simulink model "pipe_strat_enhanced"  (R2018b)
settings: Solver=VariableStepAuto  StartTime=0.0  StopTime=10.0  RelTol=1e-3
undefined symbols (not defined in the file): nodes
libraries: simulink x5, carnot x1
settings Model: Creator=jonas.gottschald  LastModifiedBy=P41573
settings DataIOCC: ReturnWorkspaceOutputs=on

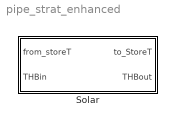
== system pipe_strat_enhanced ==
  Solar : Subsystem  AncestorBlock=carnot/Storage/Thermal/Storage_Ports/Pipe_stratified  mask(pipe connection to storage){h_in=1, h_strat=0.16, h_out=0, hgt=1, dia=0.08, height=-1, nodes=nodes}
      mask prompts: h_in "relative height of the starting point of the stratification device"; h_strat "relative height of the end point of the stratification device"; h_out "relative height of outlet"; hgt "Height of storage in m"; dia "Diameter of pipe in m"; height "Height difference inlet-outlet"; nodes "Number of nodes (DO NOT CHANGE)"
      mask help:
      | The block transforms the incoming THV vector to a vector which the storage interprets as a flow into the storage fluid.
      | Give inlet- and outlet-height as a relative position from 0 (= bottom) to 1 (= top).
      mask init:
      | in = zeros(nodes,1);    % vector of length nodes
      | up = in;                % vector of length nodes
      | down = in;              % vector of length nodes
      | 
      | h_in = max(0,min(h_in,1));     % no nodes below 0 and above 1
      | h_out = max(0,min(h_out,1));   % no nodes below 0 and above 1
      | h_strat = max(0,min(h_strat,1));   % no nodes below 0 and above 1
      | set_param(gcb,'height',num2str((h_out-h_in)*hgt));
      | 
      | inlet = max(ceil(h_in*nodes),1);    % inlet position
      | outlet = max(ceil(h_out*nodes),1);  % outlet position
      | strat = max(ceil(h_strat*nodes),1);  % startification position
      | hgt = (h_out-h_in)*hgt;
      | in(inlet)=1;
      | 
      | idx_in_out = inlet:outlet;
      | if (inlet < outlet && strat < outlet && inlet < strat)      % if outlet above inlet and stratification and inlet below stratification
      |     up(inlet:outlet-1)=1;       % upwards
      |     n_concerned = inlet:strat;
      | end
      | 
      | if (inlet < outlet && strat < outlet && inlet > strat) % if outlet above inlet and stratification and inlet above stratification
      |     up(strat:outlet-1)=1;       % upwards
      |     n_concerned = strat:inlet;
      | end
      | 
      | if (inlet < outlet && strat > outlet)                  % if outlet above inlet and below stratification
      |     up(inlet:outlet-1)=1;       % upwards and
      |     down(outlet:strat-1)=1;     % downwards
      |     n_concerned = inlet:strat;
      | end
      | 
      | if (inlet > outlet && strat < outlet)                  % if outlet below inlet and above stratification
      |     up(strat:outlet-1)=1;       % upwars and
      |     down(outlet:inlet-1)=1;     % downwards
      |     n_concerned = strat:inlet;
      |     idx_in_out = outlet:inlet;
      | end
      | 
      | if (inlet > outlet && inlet > strat)                    % if inlet above outlet and above stratification
      |     down(outlet:inlet-1)=1;     % downwards
      |     n_concerned = strat:inlet;                              % if inlet above outlet and below stratification
      |     idx_in_out = outlet:inlet;
      | end
      | 
      | if (inlet > outlet && inlet < strat)
      |     down(outlet:strat-1)=1;     % downwards
      |     n_concerned = inlet:strat;
      |     idx_in_out = outlet:inlet;
      | end
      mask Help: web(fullfile(path_carnot('help'),'StoragePorts_PipeConnections.html'),'-helpbrowser')
      mask TypeOptions dia: Pressure_Drop_StoragePipe/dia
      mask TypeOptions height: Pressure_Drop_StoragePipe/hgt
      mask DialogControl ParameterTabVar0 Prompt: Geometry
      mask DialogControl ParameterTabVar02 Prompt: Calculation
      mask Display: disp('Pipe STRAT')

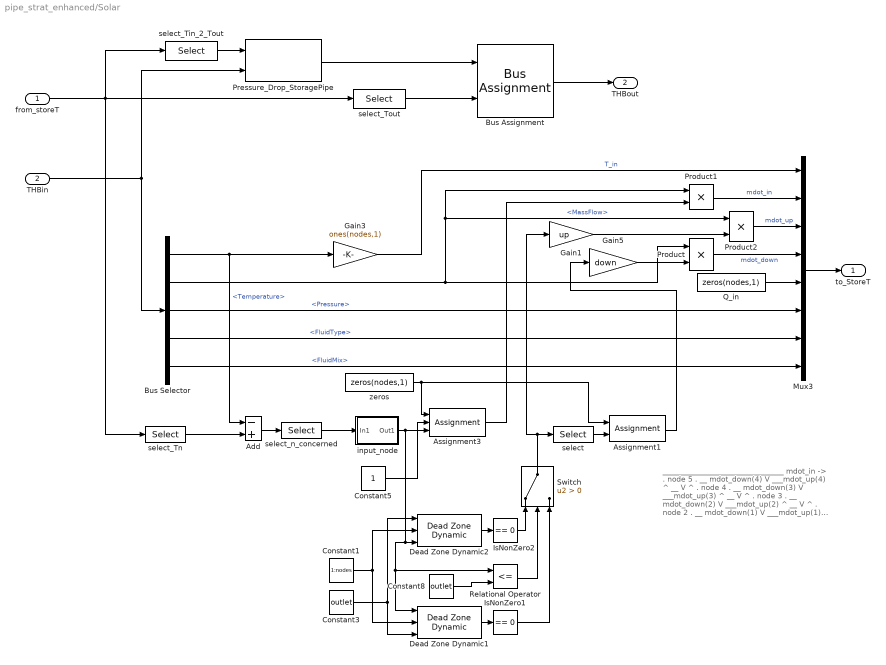
== system pipe_strat_enhanced/Solar ==
  note: _________________________________
      | mdot_in ->                                                .
      | node 5                     .
      | __ mdot_down(4) V  ___mdot_up(4) ^ __
      | V                           ^    .
      | node 4                    .
      | __ mdot_down(3) V  ___mdot_up(3) ^ __
      | V                           ^    .
      | node 3                    .
      | __ mdot_down(2) V  ___mdot_up(2) ^ __
      | V                           ^    .
      | node 2                    .
      | __ mdot_down(1) V  ___mdot_up(1) ^ __
      | V                           ^    .
      | node 1                    .
      | _________________________________
  from_storeT : Inport
  THBin : Inport  Port=2
  Add : Sum  Inputs=-+
  Assignment1 : Assignment  DiagnosticForDimensions=Warning  IndexOptions=Index vector (dialog)  Indices=1:nodes-1  OutputSizes=1
  Assignment3 : Assignment  DiagnosticForDimensions=Warning  IndexOptions=Index vector (port)  Indices=1:nodes-1  OutputSizes=1
  Bus Assignment : BusAssignment  AssignedSignals=Temperature
  Bus Selector : BusSelector  OutputSignals=Temperature,MassFlow,Pressure,FluidType,FluidMix
  Constant1 : Constant  Value=1:nodes
  Constant3 : Constant  Value=outlet
  Constant5 : Constant
  Constant8 : Constant  Value=outlet
  Dead Zone Dynamic1 : simulink/Discontinuities/Dead Zone Dynamic
      settings: SourceProductBaseCode=SL
  Dead Zone Dynamic2 : simulink/Discontinuities/Dead Zone Dynamic
      settings: SourceProductBaseCode=SL
  Gain1 : Gain  Gain=up
  Gain3 : Gain  Gain=ones(nodes,1)
  Gain5 : Gain  Gain=down
  IsNonZero1 : simulink/Logic and Bit Operations/Compare To Zero  relop===  OutDataTypeStr=boolean
  IsNonZero2 : simulink/Logic and Bit Operations/Compare To Zero  relop===  OutDataTypeStr=boolean
  Mux3 : Mux  Inputs=8
  Pressure_Drop_StoragePipe : carnot/Basic/Pressure_Drop/Pressure_Drop_StoragePipe  dpipe=0.04  dstg=1  hgt=height
      settings: SourceProductName=Carnot
  Product : Product  RndMeth=Zero
  Product1 : Product  RndMeth=Zero
  Product2 : Product  RndMeth=Zero
  Q_in : Constant  Value=zeros(nodes,1)
  Relational Operator : RelationalOperator  Operator=<=  OutDataTypeStr=boolean  RndMeth=Simplest
  Switch : Switch  Criteria=u2 > Threshold
  input_node : Subsystem
  select : Selector  InputPortWidth=nodes  IndexOptions=Index vector (dialog)  Indices=2:nodes  OutputSizes=1
  select_Tin_2_Tout : Selector  InputPortWidth=nodes  IndexOptions=Index vector (dialog)  Indices=[idx_in_out]  OutputSizes=1
  select_Tn : Selector  InputPortWidth=nodes  IndexOptions=Index vector (dialog)  Indices=[1:nodes]  OutputSizes=1
  select_Tout : Selector  InputPortWidth=nodes  IndexOptions=Index vector (dialog)  Indices=[outlet]  OutputSizes=1
  select_n_concerned : Selector  InputPortWidth=nodes  IndexOptions=Index vector (dialog)  Indices=n_concerned  OutputSizes=1
  zeros : Constant  Value=zeros(nodes,1)
  to_StoreT : Outport  VectorParamsAs1DForOutWhenUnconnected=off
  THBout : Outport  Port=2  VectorParamsAs1DForOutWhenUnconnected=off
  wires:
  select_Tin_2_Tout/1 -> Pressure_Drop_StoragePipe/1
  Pressure_Drop_StoragePipe/1 -> Bus Assignment/1
  Product1/1 -> Mux3/2  "mdot_in"
  Gain5/1 -> Product/2
  Product/1 -> Mux3/4  "mdot_down"
  from_storeT/1 -> select_Tin_2_Tout/1, select_Tn/1, select_Tout/1
  THBin/1 -> Pressure_Drop_StoragePipe/2, Bus Selector/1
  Bus Selector/4 -> Mux3/7  "<FluidType>"
  Bus Selector/3 -> Mux3/6  "<Pressure>"
  Bus Selector/2 -> Product/1, Product2/1, Product1/1  "<MassFlow>"
  Bus Selector/1 -> Gain3/1, Add/1  "<Temperature>"
  select_Tout/1 -> Bus Assignment/2
  Gain3/1 -> Mux3/1  "T_in"
  Q_in/1 -> Mux3/5
  Bus Assignment/1 -> THBout/1
  Bus Selector/5 -> Mux3/8  "<FluidMix>"
  select_Tn/1 -> Add/2
  Gain1/1 -> Product2/2
  Product2/1 -> Mux3/3  "mdot_up"
  Add/1 -> select_n_concerned/1
  Assignment3/1 -> Product1/2
  Dead Zone Dynamic1/1 -> IsNonZero1/1
  Constant8/1 -> Relational Operator/2
  Relational Operator/1 -> Switch/2
  Assignment1/1 -> Gain5/1
  select_n_concerned/1 -> input_node/1(In1)
  Switch/1 -> Gain1/1, select/1
  Mux3/1 -> to_StoreT/1
  input_node/1(Out1) -> Assignment3/3, Dead Zone Dynamic1/1, Relational Operator/1, Dead Zone Dynamic2/3
  IsNonZero1/1 -> Switch/3
  Constant3/1 -> Dead Zone Dynamic2/1, Dead Zone Dynamic1/3
  Dead Zone Dynamic2/1 -> IsNonZero2/1
  IsNonZero2/1 -> Switch/1
  select/1 -> Assignment1/2
  Constant1/1 -> Dead Zone Dynamic2/2, Dead Zone Dynamic1/2
  Constant5/1 -> Assignment3/2
  zeros/1 -> Assignment1/1, Assignment3/1

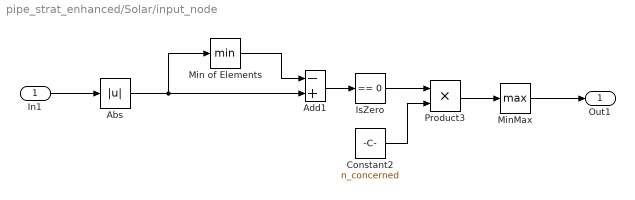
== system pipe_strat_enhanced/Solar/input_node ==
  In1 : Inport
  Abs : Abs
  Add1 : Sum  Inputs=-+
  Constant2 : Constant  Value=n_concerned
  IsZero : simulink/Logic and Bit Operations/Compare To Zero  relop===  OutDataTypeStr=boolean
  Min of Elements : MinMax
  MinMax : MinMax  Function=max
  Product3 : Product
  Out1 : Outport  VectorParamsAs1DForOutWhenUnconnected=off
  wires:
  In1/1 -> Abs/1
  Constant2/1 -> Product3/2
  IsZero/1 -> Product3/1
  Min of Elements/1 -> Add1/1
  Add1/1 -> IsZero/1
  Product3/1 -> MinMax/1
  MinMax/1 -> Out1/1
  Abs/1 -> Min of Elements/1, Add1/2
